simulink model "l1"  (R2024a)
settings: Solver=ode4  StartTime=0.0  StopTime=10.0  FixedStep=2^-7  RelTol=1e-3
libraries: simulink x1
settings Model: Creator=gm54508  LastModifiedBy=gm54508

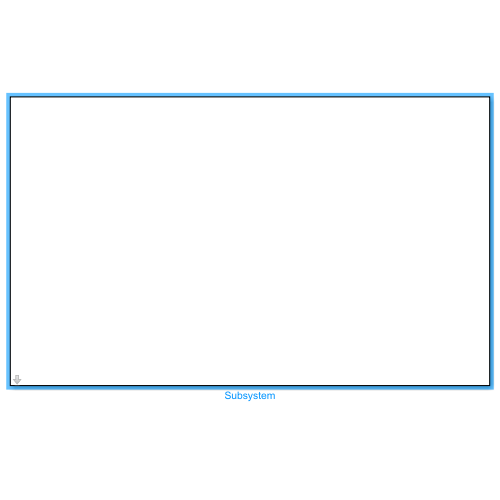
[thumbnail: Simulink's stored preview of the top-level diagram]
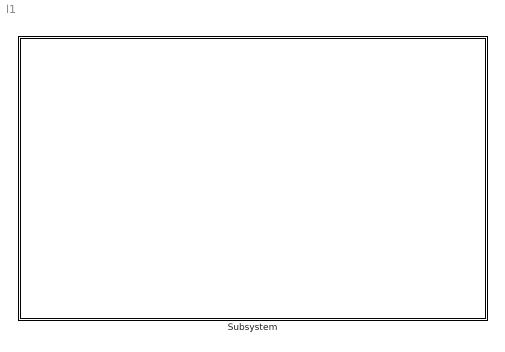
== system l1 ==
  Subsystem : Subsystem  mask{x=2, y=7, Vx=10, Vy=5, M=250, R=3, G=9.81, rs=0.2}

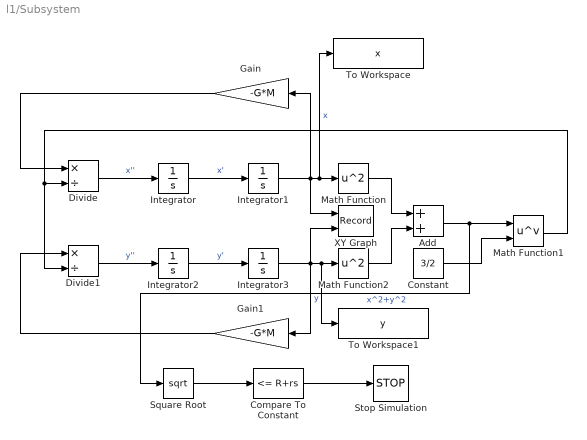
== system l1/Subsystem ==
  Add : Sum
  Compare To Constant : simulink/Logic and Bit Operations/Compare To Constant  relop=<=  const=R+rs  OutDataTypeStr=boolean
  Constant : Constant  Value=3/2
  Divide : Product  Inputs=*/
  Divide1 : Product  Inputs=*/
  Gain : Gain  Gain=-G*M
  Gain1 : Gain  Gain=-G*M
  Integrator : Integrator  InitialCondition=Vx
  Integrator1 : Integrator  InitialCondition=x
  Integrator2 : Integrator  InitialCondition=Vy
  Integrator3 : Integrator  InitialCondition=y
  Math Function : Math  Operator=square
  Math Function1 : Math  Operator=pow
  Math Function2 : Math  Operator=square
  Square Root : Sqrt
  Stop Simulation : Stop
  To Workspace : ToWorkspace  VariableName=x  SampleTime=-1
  To Workspace1 : ToWorkspace  VariableName=y  SampleTime=-1
  XY Graph : Record  FileSettingsInternal="{\"entries\":[{\"content\":{\"excelSettings\":{\"content\":{},\"type\":\"Streamout.ExcelSettings\"}},\"type\":\"Streamout.FileSettingStorage\",\"uuid\":\"\"}],\"packageUris\":[\"http:\\/\\/schema.mathworks.com\\/mf0\\/streamout_blocks\\/R2020a\"],\"version\":\"1.0\"}"  Layout=[1 1]  SignalsInternal="{\"entries\":[{\"content\":{\"signals\":[{\"content\":{\"blockPath\":[],\"dimensions\":[1],\"domain\":\"\",\"lineColor\":\"#a2142f\",\"plots\":[ 1 ],\"port\":1,\"sid\":[\"\"],\"signalID\":1,\"signalName\":\"x\"},\"type\":\"RecordBlkView.Signal\",\"uuid\":\"\"},{\"content\":{\"blockPath\":[],\"dimensions\":[1],\"domain\":\"\",\"lineColor\":\"#139fff\",\"plots\":[ 1 ],\"port\":2,\"sid\":[\"\"],\"signalID\":2,\"signalName\":\"y\"},\"type\":\"RecordBlkView.Signal\",\"uuid\":\"\"}]},\"type\":\"RecordBlkView.InputSignals\",\"uuid\":\"\"}],\"packageUris\":[\"http:\\/\\/schema.mathworks.com\\/mf0\\/streamout_blocks\\/R2020a\"],\"version\":\"1.0\"}"  VisualizationBindings="{\"xyplotplugin\":{\"info\":[{\"series\":[{\"bindingParametersList\":[{\"parameter\":\"X-Axis\",\"signalID\":1,\"signalName\":\"x\"},{\"parameter\":\"Y-Axis\",\"signalID\":2,\"signalName\":\"y\"}],\"seriesID\":0}],\"subplotID\":1}]}}"  CompatibilityTag=XY
  wires:
  Math Function2/1 -> Add/2
  Math Function1/1 -> Divide1/2, Divide/2
  Divide/1 -> Integrator/1  "x''"
  Integrator3/1 -> XY Graph/2, Gain1/1, To Workspace1/1, Math Function2/1  "y"
  Add/1 -> Square Root/1, Math Function1/1  "x^2+y^2"
  Integrator/1 -> Integrator1/1  "x'"
  Integrator2/1 -> Integrator3/1  "y'"
  Math Function/1 -> Add/1
  Divide1/1 -> Integrator2/1  "y''"
  Constant/1 -> Math Function1/2
  Integrator1/1 -> XY Graph/1, Gain/1, To Workspace/1, Math Function/1  "x"
  Gain/1 -> Divide/1
  Gain1/1 -> Divide1/1
  Compare To Constant/1 -> Stop Simulation/1
  Square Root/1 -> Compare To Constant/1
